simulink model "vacuum_LQG_continuous_time"  (R2022a)
settings: Solver=VariableStepAuto  StartTime=0.0  StopTime=RunTime  FixedStep=SampleTime  RelTol=1e-3
undefined symbols (not defined in the file): K_vacuum, SampleTime, sysc_vacuum, syskf
libraries: simulink x1
settings Model: Creator=ducks  LastModifiedBy=ducks
settings DataIOCC: ExternalInput=[t,V]

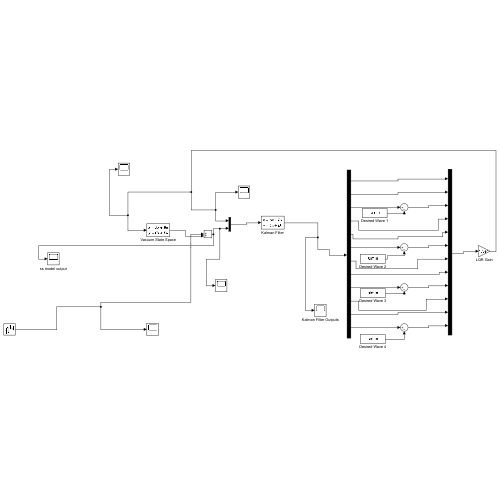
[thumbnail: Simulink's stored preview of the top-level diagram]
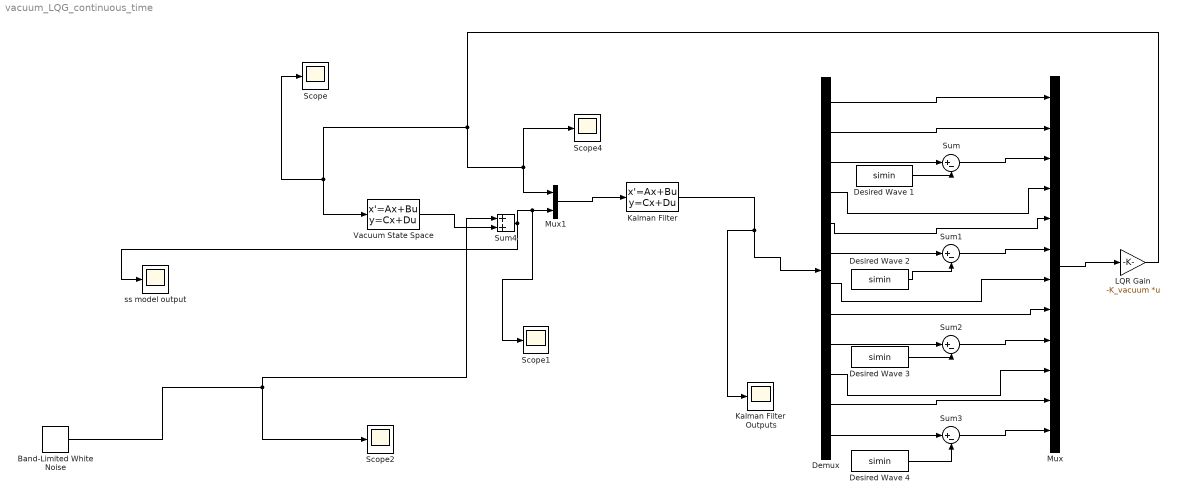
== system vacuum_LQG_continuous_time ==
  Band-Limited White Noise : simulink/Sources/Band-Limited White Noise  Cov=NoisePower  Ts=SampleTime  seed=[23341]
  Demux : Demux  Outputs=12
  Desired Wave {1..4} (4 alike) : FromWorkspace  VariableName=simin
  Kalman Filter : StateSpace  A=syskf.A  B=syskf.B  C=syskf.C  D=syskf.D  InitialCondition=0
  Kalman Filter Outputs : Scope
  LQR Gain : Gain  Gain=-K_vacuum  Multiplication=Matrix(K*u) (u vector)
  Mux : Mux  Inputs=12
  Mux1 : Mux  Inputs=2
  Scope{,1..2,4} (4 alike) : Scope
  Sum{,1..3} (4 alike) : Sum  Inputs=|+-
  Sum4 : Sum  Inputs=|++
  Vacuum State Space : StateSpace  A=sysc_vacuum.A  B=sysc_vacuum.B  C=sysc_vacuum.C  D=sysc_vacuum.D  InitialCondition=0
  ss model output : Scope
  wires:
  Desired Wave 3/1 -> Sum2/2
  Sum2/1 -> Mux/9
  Demux/1 -> Mux/1
  Kalman Filter/1 -> Kalman Filter Outputs/1, Demux/1
  Demux/7 -> Mux/7
  Demux/9 -> Sum2/1
  Demux/11 -> Mux/11
  Demux/2 -> Mux/2
  Desired Wave 2/1 -> Sum1/2
  Sum/1 -> Mux/3
  Desired Wave 1/1 -> Sum/2
  Demux/5 -> Mux/5
  Demux/12 -> Sum3/1
  Sum3/1 -> Mux/12
  Demux/3 -> Sum/1
  Desired Wave 4/1 -> Sum3/2
  Demux/8 -> Mux/8
  Demux/4 -> Mux/4
  Sum1/1 -> Mux/6
  Demux/10 -> Mux/10
  Demux/6 -> Sum1/1
  Vacuum State Space/1 -> Sum4/2
  LQR Gain/1 -> Scope4/1, Mux1/1, Vacuum State Space/1, Scope/1
  Sum4/1 -> ss model output/1, Scope1/1, Mux1/2
  Mux/1 -> LQR Gain/1
  Mux1/1 -> Kalman Filter/1
  Band-Limited White Noise/1 -> Scope2/1, Sum4/1
